simulink model "Simulation without PID"  (R2023b)
settings: Solver=VariableStepAuto  StartTime=0.0  StopTime=0.3  RelTol=1e-3
libraries: spsSeriesRLCBranchLib x10, spsDiodeLib x8, spsVoltageMeasurementLib x3, spsCurrentMeasurementLib x2, spsDCVoltageSourceLib x1, spsMosfetLib x1, sps_lib x1
settings Model: Creator=thiru  LastModifiedBy=thiru

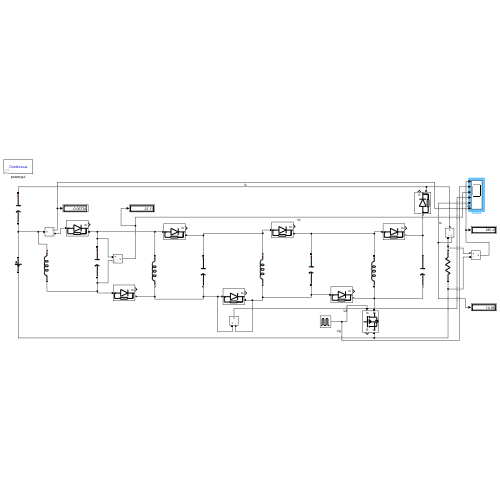
[thumbnail: Simulink's stored preview of the top-level diagram]
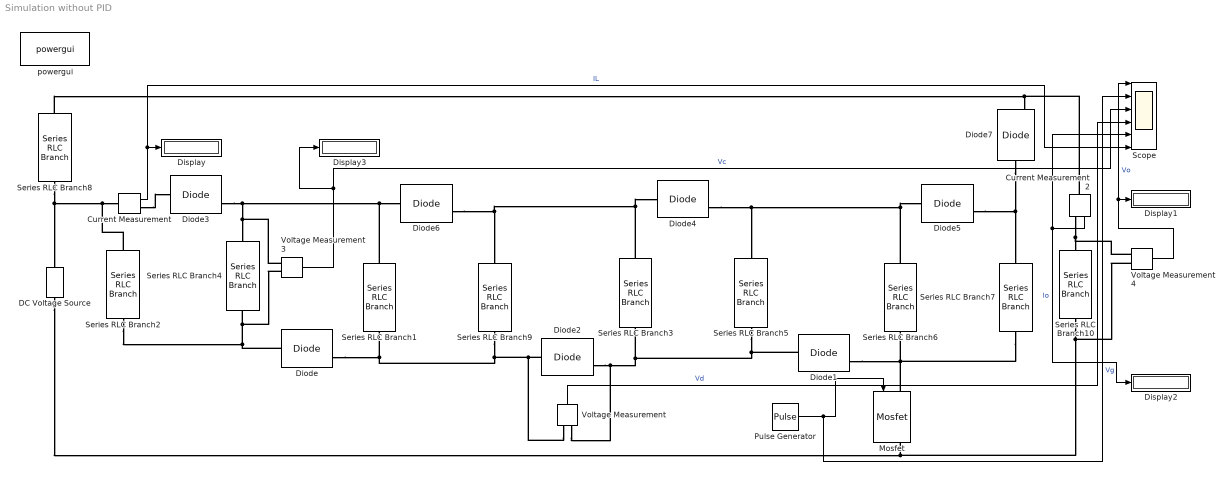
== system Simulation without PID ==
  Current Measurement : spsCurrentMeasurementLib/Current Measurement  PhasorSimulation=off  OutputType=Complex  PSBequivalent=0
  Current Measurement2 : spsCurrentMeasurementLib/Current Measurement  PhasorSimulation=off  OutputType=Complex  PSBequivalent=0
  DC Voltage Source : spsDCVoltageSourceLib/DC Voltage Source  Amplitude=50  Measurements=None
  Diode{,1..7} (8 alike) : spsDiodeLib/Diode  Ron=0.001  Lon=0  Vf=0.8  IC=0  UseSnubber=0  Rs=500  Cs=250e-9  Measurements=on
  Display{,1..3} (4 alike) : Display
  Mosfet : spsMosfetLib/Mosfet  Ron=0.1  Lon=0  Rd=0.01  Vfd=0  IC=0  Rs=1e5  Cs=inf  Measurements=on
  Pulse Generator : DiscretePulseGenerator  PulseType=Time based  Period=1/50000  PulseWidth=60
  Scope : Scope  NumInputPorts=6
  Series RLC Branch{1..3,6} (4 alike) : spsSeriesRLCBranchLib/Series RLC Branch  LConnTagsString=__new0  RConnTagsString=__new0  BranchType=L  Resistance=1  Inductance=100e-6  SetiL0=off  InitialCurrent=0  Capacitance=1e-6  Setx0=off  InitialVoltage=0  Measurements=None
  Series RLC Branch10 : spsSeriesRLCBranchLib/Series RLC Branch  LConnTagsString=__new0  RConnTagsString=__new0  BranchType=R  Resistance=20  Inductance=100e-6  SetiL0=off  InitialCurrent=0  Capacitance=1e-6  Setx0=off  InitialVoltage=0  Measurements=None
  Series RLC Branch{4..5,7..9} (5 alike) : spsSeriesRLCBranchLib/Series RLC Branch  LConnTagsString=__new0  RConnTagsString=__new0  BranchType=C  Resistance=1  Inductance=100e-6  SetiL0=off  InitialCurrent=0  Capacitance=100e-6  Setx0=off  InitialVoltage=0  Measurements=None
  Voltage Measurement : spsVoltageMeasurementLib/Voltage Measurement  PhasorSimulation=off  OutputType=Complex  PSBequivalent=0
  Voltage Measurement3 : spsVoltageMeasurementLib/Voltage Measurement  PhasorSimulation=off  OutputType=Complex  PSBequivalent=0
  Voltage Measurement4 : spsVoltageMeasurementLib/Voltage Measurement  PhasorSimulation=off  OutputType=Complex  PSBequivalent=0
  powergui : sps_lib/powergui  Priority=1  SimulationMode=Continuous  SampleTime=50e-6  frequency=60  Iterations=50  frequencyindice=0  Pbase=100e6  ErrMax=1e-4  UnitsV=kV  UnitsW=MW  buscounter=0  FunctionMessages=off  echomessages=off  EnableUseOfTLC=off  CurrentSourceSwitches=off  DisableSnubberDevices=off  DisableRonSwitches=off  DisableVfSwitches=off  DisplayEquations=off  AutomaticDiscreteSolvers=off  SolverType=Tustin/Backward Euler (TBE)  Interpol=off  ExternalGateDelay=off  methode=off  Ts=100  x0status=blocks  SPID=on  SwTol=0  HookPort=off  NonlinearTolerance=1e-4  nMaxIteration=100  ContinueOnMaxIteration=off  RestoreLinks=warning  ResistiveCurrentMeasurement=off  Frange=[0:2:500]  Ylog=off  Xlog=on  ShowGrid=off  save=off  variable=ZData  structure=0  ZoomFFT=off  StartTime=0.0  cycles=1  DisplayStyle=1  fundamental=60  FreqAxis=off  MaxFrequency=1000  frequencyindicesteady=1  RmsSteady=1  display=off
  wires:
  Pulse Generator/1 -> Scope/2, Mosfet/1  "Vg"
  Voltage Measurement4/1 -> Display1/1, Scope/1  "Vo"
  Voltage Measurement3/1 -> Display3/1, Scope/3  "Vc"
  Voltage Measurement/1 -> Scope/4  "Vd"
  Current Measurement2/1 -> Scope/5, Display2/1  "Io"
  Current Measurement/1 -> Scope/6, Display/1  "IL"
  connections:
  Series RLC Branch8/RConn1 -- DC Voltage Source/RConn1 -- Series RLC Branch2/LConn1 -- Current Measurement/LConn1
  Series RLC Branch2/RConn1 -- Diode/LConn1 -- Voltage Measurement3/LConn2 -- Series RLC Branch4/RConn1
  Current Measurement/RConn1 -- Diode3/LConn1
  Diode/RConn1 -- Voltage Measurement/LConn1 -- Diode2/LConn1 -- Series RLC Branch9/RConn1 -- Series RLC Branch1/RConn1
  Diode3/RConn1 -- Series RLC Branch1/LConn1 -- Diode6/LConn1 -- Voltage Measurement3/LConn1 -- Series RLC Branch4/LConn1
  Series RLC Branch5/RConn1 -- Diode1/LConn1 -- Voltage Measurement/LConn2 -- Diode2/RConn1 -- Series RLC Branch3/RConn1
  Diode6/RConn1 -- Series RLC Branch9/LConn1 -- Series RLC Branch3/LConn1 -- Diode4/LConn1
  Diode5/RConn1 -- Series RLC Branch7/LConn1 -- Diode7/LConn1
  Diode4/RConn1 -- Series RLC Branch5/LConn1 -- Series RLC Branch6/LConn1 -- Diode5/LConn1
  Diode1/RConn1 -- Mosfet/LConn1 -- Series RLC Branch7/RConn1 -- Series RLC Branch6/RConn1
  Series RLC Branch8/LConn1 -- Current Measurement2/LConn1 -- Diode7/RConn1
  DC Voltage Source/LConn1 -- Voltage Measurement4/LConn2 -- Series RLC Branch10/RConn1 -- Mosfet/RConn1
  Current Measurement2/RConn1 -- Voltage Measurement4/LConn1 -- Series RLC Branch10/LConn1
